simulink model "mobile_robot"  (R2022b)
settings: Solver=VariableStepAuto  StartTime=0.0  StopTime=10.0  RelTol=1e-3
settings Model: Creator=julia  LastModifiedBy=julia

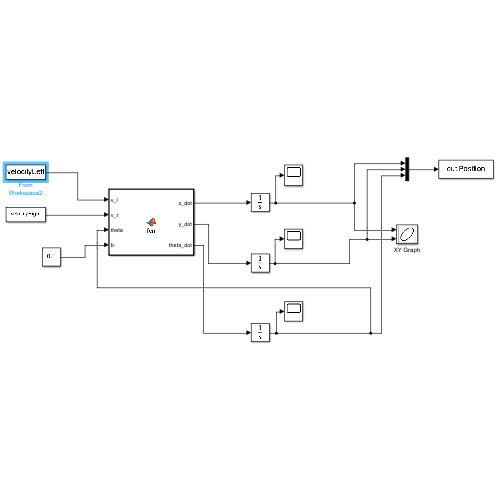
[thumbnail: Simulink's stored preview of the top-level diagram]
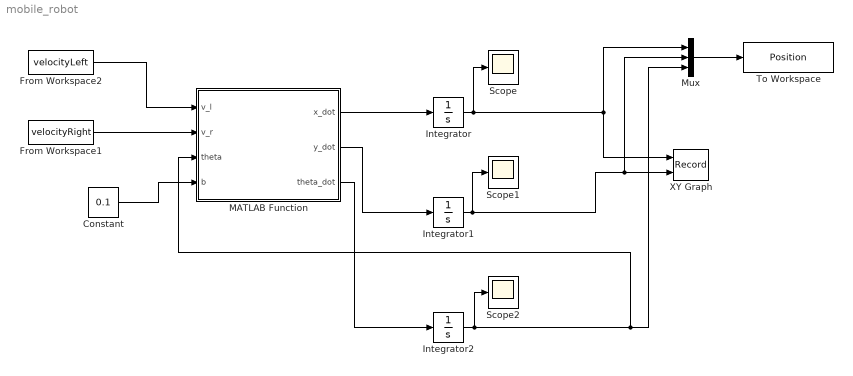
== system mobile_robot ==
  Constant : Constant  Value=0.1
  From Workspace1 : FromWorkspace  VariableName=velocityRight
  From Workspace2 : FromWorkspace  VariableName=velocityLeft
  Integrator : Integrator
  Integrator1 : Integrator
  Integrator2 : Integrator
  MATLAB Function : MATLAB Function  TreatAsAtomicUnit=on
  Mux : Mux  Inputs=3
  Scope : Scope
  Scope1 : Scope
  Scope2 : Scope
  To Workspace : ToWorkspace  VariableName=Position  SaveFormat=Timeseries  SampleTime=-1
  XY Graph : Record  FileSettingsInternal="{\"entries\":[{\"content\":{\"excelSettings\":{\"content\":{},\"type\":\"Streamout.ExcelSettings\"}},\"type\":\"Streamout.FileSettingStorage\",\"uuid\":\"ae169c74-eefd-41a2-9080-721d65abb01b\"}],\"packageUris\":[\"http://schema.mathworks.com/mf0/streamout_blocks/R2020a\"],\"version\":\"1.0\"}"  Layout=[1 1]  SignalsInternal="{\"entries\":[{\"content\":{\"signals\":[{\"content\":{\"blockPath\":[\"mobile_robot/XY Graph\"],\"channel\":[],\"dimensions\":[1],\"domain\":\"mobile_robot/XY Graph\",\"lineColor\":\"#a2142f\",\"plots\":[1],\"port\":1,\"sid\":[\"\"],\"signalID\":48,\"signalName\":\"Integrator\"},\"type\":\"RecordBlkView.Signal\",\"uuid\":\"e0bec9a0-a5f7-4d7f-8c86-236a125778a3\"},{\"content\":{\"blockPath\":[\"mobile_robot/XY Graph\"],\"channel\":[],\"dimensions\":[1],\"domain\":\"mobile_robot/XY Graph\",\"lineColor\":\"#139fff\",\"plots\":[1],\"port\":2,\"sid\":[\"\"],\"signalID\":52,\"signalName\":\"Integrator1\"},\"type\":\"RecordBlkView.Signal\",\"uuid\":\"1e5f25db-4827-4ae4-99d4-06cb38ea3cf6\"}]},\"type\":\"RecordBlkView.InputSignals\",\"uuid\":\"ee73c056-ce08-4d5e-9f9a-e37e0d821e69\"}],\"packageUris\":[\"http://schema.mathworks.com/mf0/streamout_blocks/R2020a\"],\"version\":\"1.0\"}"  VisualizationBindings="{\"xyplotplugin\":{\"info\":[{\"series\":[{\"bindingParametersList\":[{\"parameter\":\"X-Axis\",\"signalID\":48,\"signalName\":\"Integrator\"},{\"parameter\":\"Y-Axis\",\"signalID\":52,\"signalName\":\"Integrator1\"}],\"seriesID\":43101}],\"subplotID\":1}]}}"  CompatibilityTag=XY
  wires:
  From Workspace2/1 -> MATLAB Function/1(v_l)
  From Workspace1/1 -> MATLAB Function/2(v_r)
  MATLAB Function/1(x_dot) -> Integrator/1
  MATLAB Function/3(theta_dot) -> Integrator2/1
  MATLAB Function/2(y_dot) -> Integrator1/1
  Mux/1 -> To Workspace/1
  Constant/1 -> MATLAB Function/4(b)
  Integrator/1 -> Scope/1, XY Graph/1, Mux/1
  Integrator1/1 -> Scope1/1, Mux/2, XY Graph/2
  Integrator2/1 -> Scope2/1, MATLAB Function/3(theta), Mux/3

== matlab function mobile_robot/MATLAB Function ==
  data: v_l input; x_dot output; v_r input; theta input; b input; y_dot output; theta_dot output
function [x_dot, y_dot, theta_dot]  = fcn(v_l, v_r, theta, b)

x_dot = cos(theta)*(v_l+v_r)/2;
y_dot = sin(theta)*(v_l+v_r)/2;
theta_dot = (v_r-v_l)/b;

end
